simulink model "AESModel_"  (R2021a)
settings: Solver=VariableStepAuto  StartTime=0.0  StopTime=10.0  RelTol=1e-3
libraries: commrandsrc3 x2
settings Model: Creator=Vince  LastModifiedBy=Vince

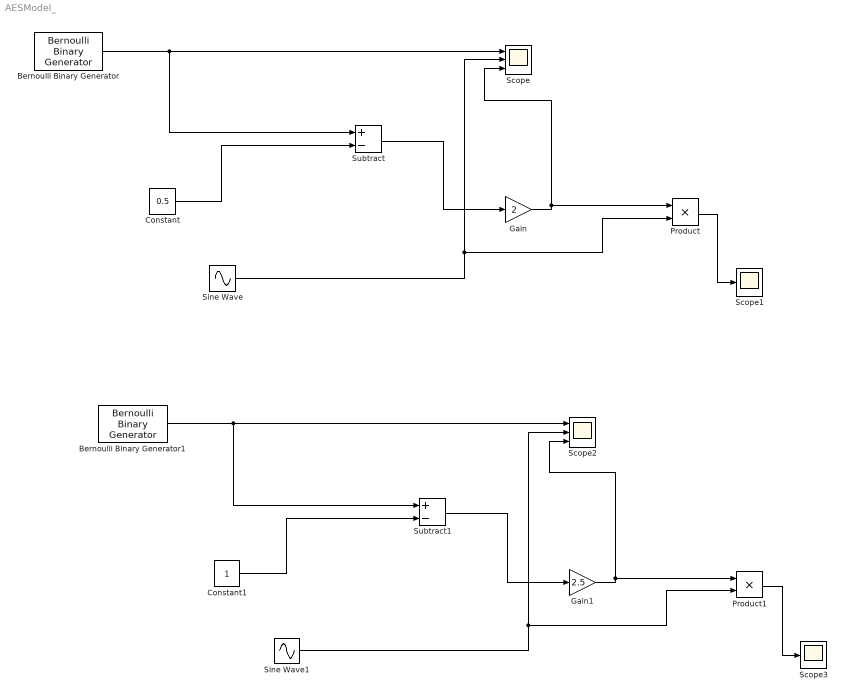
== system AESModel_ ==
  Bernoulli Binary Generator : commrandsrc3/Bernoulli Binary Generator  ProbabilityOfZero=0.5  SeedSource=Auto  Seed=0  SampleTime=1  SamplesPerFrame=1  OutputDataType=double  SimulateUsing=Interpreted execution
  Bernoulli Binary Generator1 : commrandsrc3/Bernoulli Binary Generator  ProbabilityOfZero=0.5  SeedSource=Auto  Seed=0  SampleTime=1  SamplesPerFrame=1  OutputDataType=double  SimulateUsing=Interpreted execution
  Constant : Constant  Value=0.5
  Constant1 : Constant
  Gain : Gain  Gain=2
  Gain1 : Gain  Gain=2.5
  Product : Product
  Product1 : Product
  Scope : Scope  NumInputPorts=3
  Scope1 : Scope
  Scope2 : Scope  NumInputPorts=3
  Scope3 : Scope
  Sine Wave : Sin  Frequency=4*pi  Phase=1/3200*pi  SampleTime=0
  Sine Wave1 : Sin  Frequency=4*pi  Phase=1/3200  SampleTime=0
  Subtract : Sum  Inputs=+-
  Subtract1 : Sum  Inputs=+-
  wires:
  Bernoulli Binary Generator/1 -> Subtract/1, Scope/1
  Sine Wave/1 -> Product/2, Scope/2
  Constant/1 -> Subtract/2
  Subtract/1 -> Gain/1
  Gain/1 -> Scope/3, Product/1
  Product/1 -> Scope1/1
  Bernoulli Binary Generator1/1 -> Subtract1/1, Scope2/1
  Product1/1 -> Scope3/1
  Subtract1/1 -> Gain1/1
  Sine Wave1/1 -> Product1/2, Scope2/2
  Gain1/1 -> Scope2/3, Product1/1
  Constant1/1 -> Subtract1/2
